simulink model "Doppelpendel_EKF_2015a"  (R2015a)
settings: Solver=ode45  StartTime=0.0  StopTime=10
undefined symbols (not defined in the file or in its folder): parDP, parEKF, parLQR
libraries: cstblocks x3
(part 2 of 2)

== matlab function Doppelpendel_EKF_2015a/Regler/LQR+EKF ==
  settings: updateMethod=DISCRETE  sampleTime=parLQR.Ta
  data: Switch_Rueckfuehrung input; statesd input; states input; uFF input; uG output; parDP parameter; parLQR parameter; parEKF parameter; xestout output; e_phi1 output; e_s output; e output; Pplus output
function [uG,xestout,e_phi1,e_s,e,Pplus]  = LQG(Switch_Rueckfuehrung,statesd,states,uFF,parDP,parLQR,parEKF)

%Anfangsbedinungen = Ruhelagen
persistent xI
if isempty(xI)
    xI = double(0);
end

persistent xminus
if isempty(xminus)
    xminus = [parEKF.phi10;parEKF.omega10;parEKF.phi20;parEKF.omega20;parEKF.s0;parEKF.w0];
end

persistent Pminus
if isempty( Pminus) 
    Pminus = diag([parEKF.delta,parEKF.delta,parEKF.delta,parEKF.delta,parEKF.delta,parEKF.delta]); 
end

%Ausgang
xestout=xminus;

%Beobachterrückführung ein/aus
if (Switch_Rueckfuehrung)
    xest=xestout;
else
    xest=states;
end

%%%%%%%%%%%%%%%%%%%%%%%%%%%%%%%%%%%%%%%%%%%%%%%%%%%%%%%%%%%%%%%%%%%%%%%%%%%
%LQR-Regler
%%%%%%%%%%%%%%%%%%%%%%%%%%%%%%%%%%%%%%%%%%%%%%%%%%%%%%%%%%%%%%%%%%%%%%%%%%%

% Folgendes hier bitte ausführen:
% 1.) PI-Zustandsregler einfügen

% xI(k+1) = xI(k) + (yd - y) (xI = eI)
xI = xI + (statesd(5) - xest(5));


% 2.) if (reset_cont==1) xI=0 end
% if (reset_cont==1)
%     xI=0;
% end

%Gesamtrückführung
% uFB = [kxT kI] [delta_e; delta_eI] (2.26b)
uG = parLQR.kx*(xest - statesd) + parLQR.kI * xI + uFF;

%%%%%%%%%%%%%%%%%%%%%%%%%%%%%%%%%%%%%%%%%%%%%%%%%%%%%%%%%%%%%%%%%%%%%%%%%%%
%EKF
%%%%%%%%%%%%%%%%%%%%%%%%%%%%%%%%%%%%%%%%%%%%%%%%%%%%%%%%%%%%%%%%%%%%%%%%%%%

% Folgendes hier bitte ausführen:
% 1.) Extended-Kalman-Filter einfügen

Ck = [0 0 0 0 1 0; 1 0 0 0 0 0];
% Hk = 0;
Lk_dach = Pminus*Ck' / (Ck*Pminus*Ck' + parEKF.Rn);

xplus = xminus + Lk_dach*( [states(5); states(1)] - [ xest(5); xest(1)] );
Pplus = (eye(6) - Lk_dach*Ck) * Pminus;

Phi_k = eye(6) + parDP.Ta*fcnAsys(xplus,uG,parDP);
Gk = eye(6);

xminus = xplus + parDP.Ta*fcnfx(xplus,uG,parDP);
Pminus = Phi_k*Pplus*Phi_k' + Gk*parEKF.Qn*Gk';

e_phi1 = states(1) - xminus(1);
e_s = states(5)- xminus(5);
e = 0;

end

%% Rechte Seite
function fx = fcnfx(xplus,uG,parDP)

InvD11 = parDP.m2*parDP.a2*parDP.a2+parDP.J2;
InvD12 = -parDP.m2*parDP.l1*parDP.a2*cos(xplus(1)-xplus(3));
InvD22 = parDP.J1+parDP.a1*parDP.a1*parDP.m1+parDP.m2*parDP.l1*parDP.l1;
den    = (parDP.J1+parDP.a1*parDP.a1*parDP.m1+parDP.m2*parDP.l1*parDP.l1)*(parDP.m2*parDP.a2*parDP.a2+parDP.J2)-parDP.m2*parDP.m2*parDP.l1*parDP.l1*parDP.a2*parDP.a2*(cos(xplus(1)-xplus(3)))^2;
gg1    = parDP.d2*xplus(2)-parDP.d2*xplus(4)-parDP.m2*parDP.l1*cos(xplus(1))*uG-parDP.m1*parDP.g*parDP.a1*sin(xplus(1))-parDP.m2*parDP.g*parDP.l1*sin(xplus(1))-parDP.m1*parDP.a1*cos(xplus(1))*uG+parDP.d1*xplus(2)+parDP.m2*parDP.l1*parDP.a2*xplus(4)*xplus(4)*sin(xplus(1)-xplus(3));
gg2    = -parDP.m2*parDP.g*parDP.a2*sin(xplus(3))-parDP.m2*parDP.a2*cos(xplus(3))*uG-parDP.m2*parDP.a2*parDP.l1*xplus(2)*xplus(2)*sin(xplus(1)-xplus(3))+parDP.d2*xplus(4)-parDP.d2*xplus(2);

fx = [xplus(2);
    -1/den*(InvD11*gg1+InvD12*gg2);
    xplus(4);
    -1/den*(InvD12*gg1+InvD22*gg2);
    xplus(6);
    uG];

end
%% linearisierte Systemmatrix

function Asyslin = fcnAsys(xplus,u,parDP) %% linearisierte Systemmatrix

Asyslin = [0 1 0 0 0 0;
    -0.1e1 / (parDP.J1 * parDP.m2 * parDP.a2 ^ 2 + parDP.J1 * parDP.J2 + parDP.a1 ^ 2 * parDP.m1 * parDP.m2 * parDP.a2 ^ 2 + parDP.a1 ^ 2 * parDP.m1 * parDP.J2 + parDP.m2 ^ 2 * parDP.l1 ^ 2 * parDP.a2 ^ 2 + parDP.m2 * parDP.l1 ^ 2 * parDP.J2 - parDP.m2 ^ 2 * parDP.l1 ^ 2 * parDP.a2 ^ 2 * cos(xplus(1)) ^ 2 * cos(xplus(3)) ^ 2 - 0.2e1 * parDP.m2 ^ 2 * parDP.l1 ^ 2 * parDP.a2 ^ 2 * cos(xplus(1)) * cos(xplus(3)) * sin(xplus(1)) * sin(xplus(3)) - parDP.m2 ^ 2 * parDP.l1 ^ 2 * parDP.a2 ^ 2 * sin(xplus(1)) ^ 2 * sin(xplus(3)) ^ 2) ^ 2 * (-parDP.d2 * xplus(2) * parDP.m2 * parDP.a2 ^ 2 + parDP.d2 * xplus(4) * parDP.m2 * parDP.a2 ^ 2 - parDP.d1 * xplus(2) * parDP.m2 * parDP.a2 ^ 2 + parDP.m2 ^ 2 * parDP.a2 ^ 3 * sin(xplus(3)) * xplus(4) * parDP.l1 * cos(xplus(1)) * xplus(2) - parDP.m2 ^ 2 * parDP.a2 ^ 3 * cos(xplus(3)) * xplus(4) * parDP.l1 * sin(xplus(1)) * xplus(2) + parDP.m1 * parDP.a1 * sin(xplus(1)) * xplus(2) * xplus(6) * parDP.m2 * parDP.a2 ^ 2 - parDP.m2 ^ 2 * parDP.l1 * parDP.a2 ^ 2 * cos(xplus(1)) * cos(xplus(3)) * parDP.g * sin(xplus(3)) - parDP.m2 ^ 2 * parDP.l1 * parDP.a2 ^ 2 * sin(xplus(1)) * sin(xplus(3)) ^ 2 * xplus(4) * xplus(6) - parDP.m2 ^ 2 * parDP.l1 * parDP.a2 ^ 2 * sin(xplus(1)) * sin(xplus(3)) * cos(xplus(3)) * u + parDP.m2 * parDP.l1 * parDP.a2 * cos(xplus(1)) * cos(xplus(3)) * parDP.d2 * xplus(4) - parDP.m2 * parDP.l1 * parDP.a2 * cos(xplus(1)) * cos(xplus(3)) * parDP.d2 * xplus(2) + parDP.m2 * parDP.l1 * parDP.a2 * sin(xplus(1)) * sin(xplus(3)) * parDP.d2 * xplus(4) - parDP.m2 * parDP.l1 * parDP.a2 * sin(xplus(1)) * sin(xplus(3)) * parDP.d2 * xplus(2) + parDP.m2 ^ 2 * parDP.l1 * cos(xplus(1)) * u * parDP.a2 ^ 2 + parDP.m2 * parDP.l1 * cos(xplus(1)) * u * parDP.J2 + parDP.m1 * parDP.g * parDP.a1 * sin(xplus(1)) * parDP.J2 + parDP.m2 ^ 2 * parDP.g * parDP.l1 * sin(xplus(1)) * parDP.a2 ^ 2 + parDP.m2 * parDP.g * parDP.l1 * sin(xplus(1)) * parDP.J2 + parDP.m1 * parDP.a1 * cos(xplus(1)) * u * parDP.J2 + parDP.m1 * parDP.g * parDP.a1 * sin(xplus(1)) * parDP.m2 * parDP.a2 ^ 2 + parDP.m1 * parDP.a1 * cos(xplus(1)) * u * parDP.m2 * parDP.a2 ^ 2 + parDP.m1 * parDP.a1 * sin(xplus(1)) * xplus(2) * xplus(6) * parDP.J2 + parDP.m2 ^ 2 * parDP.l1 * sin(xplus(1)) * xplus(2) * xplus(6) * parDP.a2 ^ 2 + parDP.m2 * parDP.l1 * sin(xplus(1)) * xplus(2) * xplus(6) * parDP.J2 - parDP.m2 ^ 2 * parDP.l1 * parDP.a2 ^ 2 * cos(xplus(1)) * cos(xplus(3)) ^ 2 * u - parDP.m2 ^ 2 * parDP.l1 * parDP.a2 ^ 2 * sin(xplus(1)) * sin(xplus(3)) ^ 2 * parDP.g - parDP.d2 * xplus(2) * parDP.J2 - parDP.d1 * xplus(2) * parDP.J2 + parDP.d2 * xplus(4) * parDP.J2 + parDP.m2 ^ 2 * parDP.l1 ^ 2 * parDP.a2 ^ 2 * cos(xplus(1)) ^ 2 * cos(xplus(3)) * sin(xplus(3)) * xplus(4) * xplus(2) + parDP.m2 ^ 2 * parDP.l1 ^ 2 * parDP.a2 ^ 2 * sin(xplus(1)) * sin(xplus(3)) ^ 2 * xplus(4) * cos(xplus(1)) * xplus(2) - parDP.m2 ^ 2 * parDP.l1 ^ 2 * parDP.a2 ^ 2 * sin(xplus(1)) ^ 2 * sin(xplus(3)) * cos(xplus(3)) * xplus(4) * xplus(2) - parDP.m2 ^ 2 * parDP.l1 ^ 2 * parDP.a2 ^ 2 * cos(xplus(1)) * cos(xplus(3)) ^ 2 * xplus(4) * sin(xplus(1)) * xplus(2) + parDP.m2 * parDP.a2 * sin(xplus(3)) * xplus(4) * parDP.l1 * cos(xplus(1)) * xplus(2) * parDP.J2 - parDP.m2 * parDP.a2 * cos(xplus(3)) * xplus(4) * parDP.l1 * sin(xplus(1)) * xplus(2) * parDP.J2 - parDP.m2 ^ 2 * parDP.l1 * parDP.a2 ^ 2 * cos(xplus(1)) * cos(xplus(3)) * sin(xplus(3)) * xplus(4) * xplus(6)) * (0.2e1 * parDP.m2 ^ 2 * parDP.l1 ^ 2 * parDP.a2 ^ 2 * cos(xplus(1)) * cos(xplus(3)) ^ 2 * sin(xplus(1)) + 0.2e1 * parDP.m2 ^ 2 * parDP.l1 ^ 2 * parDP.a2 ^ 2 * sin(xplus(1)) ^ 2 * cos(xplus(3)) * sin(xplus(3)) - 0.2e1 * parDP.m2 ^ 2 * parDP.l1 ^ 2 * parDP.a2 ^ 2 * cos(xplus(1)) ^ 2 * cos(xplus(3)) * sin(xplus(3)) - 0.2e1 * parDP.m2 ^ 2 * parDP.l1 ^ 2 * parDP.a2 ^ 2 * sin(xplus(1)) * sin(xplus(3)) ^ 2 * cos(xplus(1))) + 0.1e1 / (parDP.J1 * parDP.m2 * parDP.a2 ^ 2 + parDP.J1 * parDP.J2 + parDP.a1 ^ 2 * parDP.m1 * parDP.m2 * parDP.a2 ^ 2 + parDP.a1 ^ 2 * parDP.m1 * parDP.J2 + parDP.m2 ^ 2 * parDP.l1 ^ 2 * parDP.a2 ^ 2 + parDP.m2 * parDP.l1 ^ 2 * parDP.J2 - parDP.m2 ^ 2 * parDP.l1 ^ 2 * parDP.a2 ^ 2 * cos(xplus(1)) ^ 2 * cos(xplus(3)) ^ 2 - 0.2e1 * parDP.m2 ^ 2 * parDP.l1 ^ 2 * parDP.a2 ^ 2 * cos(xplus(1)) * cos(xplus(3)) * sin(xplus(1)) * sin(xplus(3)) - parDP.m2 ^ 2 * parDP.l1 ^ 2 * parDP.a2 ^ 2 * sin(xplus(1)) ^ 2 * sin(xplus(3)) ^ 2) * (-parDP.m2 ^ 2 * parDP.a2 ^ 3 * sin(xplus(3)) * xplus(4) * parDP.l1 * sin(xplus(1)) * xplus(2) - parDP.m2 ^ 2 * parDP.a2 ^ 3 * cos(xplus(3)) * xplus(4) * parDP.l1 * cos(xplus(1)) * xplus(2) + parDP.m1 * parDP.a1 * cos(xplus(1)) * xplus(2) * xplus(6) * parDP.m2 * parDP.a2 ^ 2 + parDP.m2 ^ 2 * parDP.l1 * parDP.a2 ^ 2 * sin(xplus(1)) * cos(xplus(3)) * parDP.g * sin(xplus(3)) - parDP.m2 ^ 2 * parDP.l1 * parDP.a2 ^ 2 * cos(xplus(1)) * sin(xplus(3)) ^ 2 * xplus(4) * xplus(6) - parDP.m2 ^ 2 * parDP.l1 * sin(xplus(1)) * u * parDP.a2 ^ 2 - parDP.m2 ^ 2 * parDP.l1 * parDP.a2 ^ 2 * cos(xplus(1)) * sin(xplus(3)) * cos(xplus(3)) * u - parDP.m2 * parDP.l1 * parDP.a2 * sin(xplus(1)) * cos(xplus(3)) * parDP.d2 * xplus(4) + parDP.m2 * parDP.l1 * parDP.a2 * sin(xplus(1)) * cos(xplus(3)) * parDP.d2 * xplus(2) + parDP.m2 * parDP.l1 * parDP.a2 * cos(xplus(1)) * sin(xplus(3)) * parDP.d2 * xplus(4) - parDP.m2 * parDP.l1 * parDP.a2 * cos(xplus(1)) * sin(xplus(3)) * parDP.d2 * xplus(2) - parDP.m2 ^ 2 * parDP.l1 ^ 2 * parDP.a2 ^ 2 * sin(xplus(1)) ^ 2 * sin(xplus(3)) ^ 2 * xplus(4) * xplus(2) + parDP.m2 ^ 2 * parDP.l1 ^ 2 * parDP.a2 ^ 2 * sin(xplus(1)) ^ 2 * cos(xplus(3)) ^ 2 * xplus(4) * xplus(2) + parDP.m1 * parDP.g * parDP.a1 * cos(xplus(1)) * parDP.m2 * parDP.a2 ^ 2 - parDP.m1 * parDP.a1 * sin(xplus(1)) * u * parDP.m2 * parDP.a2 ^ 2 + parDP.m1 * parDP.a1 * cos(xplus(1)) * xplus(2) * xplus(6) * parDP.J2 + parDP.m2 ^ 2 * parDP.l1 * cos(xplus(1)) * xplus(2) * xplus(6) * parDP.a2 ^ 2 + parDP.m2 * parDP.l1 * cos(xplus(1)) * xplus(2) * xplus(6) * parDP.J2 + parDP.m2 ^ 2 * parDP.l1 * parDP.a2 ^ 2 * sin(xplus(1)) * cos(xplus(3)) ^ 2 * u - parDP.m2 ^ 2 * parDP.l1 * parDP.a2 ^ 2 * cos(xplus(1)) * sin(xplus(3)) ^ 2 * parDP.g - parDP.m2 * parDP.l1 * sin(xplus(1)) * u * parDP.J2 + parDP.m1 * parDP.g * parDP.a1 * cos(xplus(1)) * parDP.J2 + parDP.m2 ^ 2 * parDP.g * parDP.l1 * cos(xplus(1)) * parDP.a2 ^ 2 + parDP.m2 * parDP.g * parDP.l1 * cos(xplus(1)) * parDP.J2 - parDP.m1 * parDP.a1 * sin(xplus(1)) * u * parDP.J2 - 0.4e1 * parDP.m2 ^ 2 * parDP.l1 ^ 2 * parDP.a2 ^ 2 * cos(xplus(1)) * cos(xplus(3)) * sin(xplus(3)) * xplus(4) * xplus(2) * sin(xplus(1)) + parDP.m2 ^ 2 * parDP.l1 ^ 2 * parDP.a2 ^ 2 * cos(xplus(1)) ^ 2 * sin(xplus(3)) ^ 2 * xplus(4) * xplus(2) - parDP.m2 ^ 2 * parDP.l1 ^ 2 * parDP.a2 ^ 2 * cos(xplus(1)) ^ 2 * cos(xplus(3)) ^ 2 * xplus(4) * xplus(2) - parDP.m2 * parDP.a2 * sin(xplus(3)) * xplus(4) * parDP.l1 * sin(xplus(1)) * xplus(2) * parDP.J2 - parDP.m2 * parDP.a2 * cos(xplus(3)) * xplus(4) * parDP.l1 * cos(xplus(1)) * xplus(2) * parDP.J2 + parDP.m2 ^ 2 * parDP.l1 * parDP.a2 ^ 2 * sin(xplus(1)) * cos(xplus(3)) * sin(xplus(3)) * xplus(4) * xplus(6)) 0.1e1 / (parDP.J1 * parDP.m2 * parDP.a2 ^ 2 + parDP.J1 * parDP.J2 + parDP.a1 ^ 2 * parDP.m1 * parDP.m2 * parDP.a2 ^ 2 + parDP.a1 ^ 2 * parDP.m1 * parDP.J2 + parDP.m2 ^ 2 * parDP.l1 ^ 2 * parDP.a2 ^ 2 + parDP.m2 * parDP.l1 ^ 2 * parDP.J2 - parDP.m2 ^ 2 * parDP.l1 ^ 2 * parDP.a2 ^ 2 * cos(xplus(1)) ^ 2 * cos(xplus(3)) ^ 2 - 0.2e1 * parDP.m2 ^ 2 * parDP.l1 ^ 2 * parDP.a2 ^ 2 * cos(xplus(1)) * cos(xplus(3)) * sin(xplus(1)) * sin(xplus(3)) - parDP.m2 ^ 2 * parDP.l1 ^ 2 * parDP.a2 ^ 2 * sin(xplus(1)) ^ 2 * sin(xplus(3)) ^ 2) * (-parDP.d2 * parDP.m2 * parDP.a2 ^ 2 - parDP.d1 * parDP.m2 * parDP.a2 ^ 2 + parDP.m2 ^ 2 * parDP.a2 ^ 3 * sin(xplus(3)) * xplus(4) * parDP.l1 * cos(xplus(1)) - parDP.m2 ^ 2 * parDP.a2 ^ 3 * cos(xplus(3)) * xplus(4) * parDP.l1 * sin(xplus(1)) + parDP.m1 * parDP.a1 * sin(xplus(1)) * xplus(6) * parDP.m2 * parDP.a2 ^ 2 - parDP.m2 * parDP.l1 * parDP.a2 * cos(xplus(1)) * cos(xplus(3)) * parDP.d2 - parDP.m2 * parDP.l1 * parDP.a2 * sin(xplus(1)) * sin(xplus(3)) * parDP.d2 + parDP.m1 * parDP.a1 * sin(xplus(1)) * xplus(6) * parDP.J2 + parDP.m2 ^ 2 * parDP.l1 * sin(xplus(1)) * xplus(6) * parDP.a2 ^ 2 + parDP.m2 * parDP.l1 * sin(xplus(1)) * xplus(6) * parDP.J2 - parDP.d2 * parDP.J2 - parDP.d1 * parDP.J2 + parDP.m2 ^ 2 * parDP.l1 ^ 2 * parDP.a2 ^ 2 * cos(xplus(1)) ^ 2 * cos(xplus(3)) * sin(xplus(3)) * xplus(4) + parDP.m2 ^ 2 * parDP.l1 ^ 2 * parDP.a2 ^ 2 * sin(xplus(1)) * sin(xplus(3)) ^ 2 * xplus(4) * cos(xplus(1)) - parDP.m2 ^ 2 * parDP.l1 ^ 2 * parDP.a2 ^ 2 * sin(xplus(1)) ^ 2 * sin(xplus(3)) * cos(xplus(3)) * xplus(4) - parDP.m2 ^ 2 * parDP.l1 ^ 2 * parDP.a2 ^ 2 * cos(xplus(1)) * cos(xplus(3)) ^ 2 * xplus(4) * sin(xplus(1)) + parDP.m2 * parDP.a2 * sin(xplus(3)) * xplus(4) * parDP.l1 * cos(xplus(1)) * parDP.J2 - parDP.m2 * parDP.a2 * cos(xplus(3)) * xplus(4) * parDP.l1 * sin(xplus(1)) * parDP.J2) -0.1e1 / (parDP.J1 * parDP.m2 * parDP.a2 ^ 2 + parDP.J1 * parDP.J2 + parDP.a1 ^ 2 * parDP.m1 * parDP.m2 * parDP.a2 ^ 2 + parDP.a1 ^ 2 * parDP.m1 * parDP.J2 + parDP.m2 ^ 2 * parDP.l1 ^ 2 * parDP.a2 ^ 2 + parDP.m2 * parDP.l1 ^ 2 * parDP.J2 - parDP.m2 ^ 2 * parDP.l1 ^ 2 * parDP.a2 ^ 2 * cos(xplus(1)) ^ 2 * cos(xplus(3)) ^ 2 - 0.2e1 * parDP.m2 ^ 2 * parDP.l1 ^ 2 * parDP.a2 ^ 2 * cos(xplus(1)) * cos(xplus(3)) * sin(xplus(1)) * sin(xplus(3)) - parDP.m2 ^ 2 * parDP.l1 ^ 2 * parDP.a2 ^ 2 * sin(xplus(1)) ^ 2 * sin(xplus(3)) ^ 2) ^ 2 * (-parDP.d2 * xplus(2) * parDP.m2 * parDP.a2 ^ 2 + parDP.d2 * xplus(4) * parDP.m2 * parDP.a2 ^ 2 - parDP.d1 * xplus(2) * parDP.m2 * parDP.a2 ^ 2 + parDP.m2 ^ 2 * parDP.a2 ^ 3 * sin(xplus(3)) * xplus(4) * parDP.l1 * cos(xplus(1)) * xplus(2) - parDP.m2 ^ 2 * parDP.a2 ^ 3 * cos(xplus(3)) * xplus(4) * parDP.l1 * sin(xplus(1)) * xplus(2) + parDP.m1 * parDP.a1 * sin(xplus(1)) * xplus(2) * xplus(6) * parDP.m2 * parDP.a2 ^ 2 - parDP.m2 ^ 2 * parDP.l1 * parDP.a2 ^ 2 * cos(xplus(1)) * cos(xplus(3)) * parDP.g * sin(xplus(3)) - parDP.m2 ^ 2 * parDP.l1 * parDP.a2 ^ 2 * sin(xplus(1)) * sin(xplus(3)) ^ 2 * xplus(4) * xplus(6) - parDP.m2 ^ 2 * parDP.l1 * parDP.a2 ^ 2 * sin(xplus(1)) * sin(xplus(3)) * cos(xplus(3)) * u + parDP.m2 * parDP.l1 * parDP.a2 * cos(xplus(1)) * cos(xplus(3)) * parDP.d2 * xplus(4) - parDP.m2 * parDP.l1 * parDP.a2 * cos(xplus(1)) * cos(xplus(3)) * parDP.d2 * xplus(2) + parDP.m2 * parDP.l1 * parDP.a2 * sin(xplus(1)) * sin(xplus(3)) * parDP.d2 * xplus(4) - parDP.m2 * parDP.l1 * parDP.a2 * sin(xplus(1)) * sin(xplus(3)) * parDP.d2 * xplus(2) + parDP.m2 ^ 2 * parDP.l1 * cos(xplus(1)) * u * parDP.a2 ^ 2 + parDP.m2 * parDP.l1 * cos(xplus(1)) * u * parDP.J2 + parDP.m1 * parDP.g * parDP.a1 * sin(xplus(1)) * parDP.J2 + parDP.m2 ^ 2 * parDP.g * parDP.l1 * sin(xplus(1)) * parDP.a2 ^ 2 + parDP.m2 * parDP.g * parDP.l1 * sin(xplus(1)) * parDP.J2 + parDP.m1 * parDP.a1 * cos(xplus(1)) * u * parDP.J2 + parDP.m1 * parDP.g * parDP.a1 * sin(xplus(1)) * parDP.m2 * parDP.a2 ^ 2 + parDP.m1 * parDP.a1 * cos(xplus(1)) * u * parDP.m2 * parDP.a2 ^ 2 + parDP.m1 * parDP.a1 * sin(xplus(1)) * xplus(2) * xplus(6) * parDP.J2 + parDP.m2 ^ 2 * parDP.l1 * sin(xplus(1)) * xplus(2) * xplus(6) * parDP.a2 ^ 2 + parDP.m2 * parDP.l1 * sin(xplus(1)) * xplus(2) * xplus(6) * parDP.J2 - parDP.m2 ^ 2 * parDP.l1 * parDP.a2 ^ 2 * cos(xplus(1)) * cos(xplus(3)) ^ 2 * u - parDP.m2 ^ 2 * parDP.l1 * parDP.a2 ^ 2 * sin(xplus(1)) * sin(xplus(3)) ^ 2 * parDP.g - parDP.d2 * xplus(2) * parDP.J2 - parDP.d1 * xplus(2) * parDP.J2 + parDP.d2 * xplus(4) * parDP.J2 + parDP.m2 ^ 2 * parDP.l1 ^ 2 * parDP.a2 ^ 2 * cos(xplus(1)) ^ 2 * cos(xplus(3)) * sin(xplus(3)) * xplus(4) * xplus(2) + parDP.m2 ^ 2 * parDP.l1 ^ 2 * parDP.a2 ^ 2 * sin(xplus(1)) * sin(xplus(3)) ^ 2 * xplus(4) * cos(xplus(1)) * xplus(2) - parDP.m2 ^ 2 * parDP.l1 ^ 2 * parDP.a2 ^ 2 * sin(xplus(1)) ^ 2 * sin(xplus(3)) * cos(xplus(3)) * xplus(4) * xplus(2) - parDP.m2 ^ 2 * parDP.l1 ^ 2 * parDP.a2 ^ 2 * cos(xplus(1)) * cos(xplus(3)) ^ 2 * xplus(4) * sin(xplus(1)) * xplus(2) + parDP.m2 * parDP.a2 * sin(xplus(3)) * xplus(4) * parDP.l1 * cos(xplus(1)) * xplus(2) * parDP.J2 - parDP.m2 * parDP.a2 * cos(xplus(3)) * xplus(4) * parDP.l1 * sin(xplus(1)) * xplus(2) * parDP.J2 - parDP.m2 ^ 2 * parDP.l1 * parDP.a2 ^ 2 * cos(xplus(1)) * cos(xplus(3)) * sin(xplus(3)) * xplus(4) * xplus(6)) * (0.2e1 * parDP.m2 ^ 2 * parDP.l1 ^ 2 * parDP.a2 ^ 2 * cos(xplus(1)) ^ 2 * cos(xplus(3)) * sin(xplus(3)) + 0.2e1 * parDP.m2 ^ 2 * parDP.l1 ^ 2 * parDP.a2 ^ 2 * sin(xplus(1)) * sin(xplus(3)) ^ 2 * cos(xplus(1)) - 0.2e1 * parDP.m2 ^ 2 * parDP.l1 ^ 2 * parDP.a2 ^ 2 * cos(xplus(1)) * cos(xplus(3)) ^ 2 * sin(xplus(1)) - 0.2e1 * parDP.m2 ^ 2 * parDP.l1 ^ 2 * parDP.a2 ^ 2 * sin(xplus(1)) ^ 2 * cos(xplus(3)) * sin(xplus(3))) + 0.1e1 / (parDP.J1 * parDP.m2 * parDP.a2 ^ 2 + parDP.J1 * parDP.J2 + parDP.a1 ^ 2 * parDP.m1 * parDP.m2 * parDP.a2 ^ 2 + parDP.a1 ^ 2 * parDP.m1 * parDP.J2 + parDP.m2 ^ 2 * parDP.l1 ^ 2 * parDP.a2 ^ 2 + parDP.m2 * parDP.l1 ^ 2 * parDP.J2 - parDP.m2 ^ 2 * parDP.l1 ^ 2 * parDP.a2 ^ 2 * cos(xplus(1)) ^ 2 * cos(xplus(3)) ^ 2 - 0.2e1 * parDP.m2 ^ 2 * parDP.l1 ^ 2 * parDP.a2 ^ 2 * cos(xplus(1)) * cos(xplus(3)) * sin(xplus(1)) * sin(xplus(3)) - parDP.m2 ^ 2 * parDP.l1 ^ 2 * parDP.a2 ^ 2 * sin(xplus(1)) ^ 2 * sin(xplus(3)) ^ 2) * (parDP.m2 ^ 2 * parDP.a2 ^ 3 * cos(xplus(3)) * xplus(4) * parDP.l1 * cos(xplus(1)) * xplus(2) + parDP.m2 ^ 2 * parDP.a2 ^ 3 * sin(xplus(3)) * xplus(4) * parDP.l1 * sin(xplus(1)) * xplus(2) + parDP.m2 ^ 2 * parDP.l1 * parDP.a2 ^ 2 * cos(xplus(1)) * sin(xplus(3)) ^ 2 * parDP.g - parDP.m2 ^ 2 * parDP.l1 * parDP.a2 ^ 2 * cos(xplus(1)) * cos(xplus(3)) ^ 2 * parDP.g - 0.2e1 * parDP.m2 ^ 2 * parDP.l1 * parDP.a2 ^ 2 * sin(xplus(1)) * cos(xplus(3)) * sin(xplus(3)) * xplus(4) * xplus(6) - parDP.m2 ^ 2 * parDP.l1 * parDP.a2 ^ 2 * sin(xplus(1)) * cos(xplus(3)) ^ 2 * u + parDP.m2 ^ 2 * parDP.l1 * parDP.a2 ^ 2 * sin(xplus(1)) * sin(xplus(3)) ^ 2 * u - parDP.m2 * parDP.l1 * parDP.a2 * cos(xplus(1)) * sin(xplus(3)) * parDP.d2 * xplus(4) + parDP.m2 * parDP.l1 * parDP.a2 * cos(xplus(1)) * sin(xplus(3)) * parDP.d2 * xplus(2) + parDP.m2 * parDP.l1 * parDP.a2 * sin(xplus(1)) * cos(xplus(3)) * parDP.d2 * xplus(4) - parDP.m2 * parDP.l1 * parDP.a2 * sin(xplus(1)) * cos(xplus(3)) * parDP.d2 * xplus(2) + 0.2e1 * parDP.m2 ^ 2 * parDP.l1 * parDP.a2 ^ 2 * cos(xplus(1)) * sin(xplus(3)) * cos(xplus(3)) * u - 0.2e1 * parDP.m2 ^ 2 * parDP.l1 * parDP.a2 ^ 2 * sin(xplus(1)) * cos(xplus(3)) * parDP.g * sin(xplus(3)) - parDP.m2 ^ 2 * parDP.l1 ^ 2 * parDP.a2 ^ 2 * cos(xplus(1)) ^ 2 * sin(xplus(3)) ^ 2 * xplus(4) * xplus(2) + parDP.m2 ^ 2 * parDP.l1 ^ 2 * parDP.a2 ^ 2 * cos(xplus(1)) ^ 2 * cos(xplus(3)) ^ 2 * xplus(4) * xplus(2) + 0.4e1 * parDP.m2 ^ 2 * parDP.l1 ^ 2 * parDP.a2 ^ 2 * cos(xplus(1)) * cos(xplus(3)) * sin(xplus(3)) * xplus(4) * xplus(2) * sin(xplus(1)) - parDP.m2 ^ 2 * parDP.l1 ^ 2 * parDP.a2 ^ 2 * sin(xplus(1)) ^ 2 * cos(xplus(3)) ^ 2 * xplus(4) * xplus(2) + parDP.m2 ^ 2 * parDP.l1 ^ 2 * parDP.a2 ^ 2 * sin(xplus(1)) ^ 2 * sin(xplus(3)) ^ 2 * xplus(4) * xplus(2) + parDP.m2 * parDP.a2 * cos(xplus(3)) * xplus(4) * parDP.l1 * cos(xplus(1)) * xplus(2) * parDP.J2 + parDP.m2 * parDP.a2 * sin(xplus(3)) * xplus(4) * parDP.l1 * sin(xplus(1)) * xplus(2) * parDP.J2 + parDP.m2 ^ 2 * parDP.l1 * parDP.a2 ^ 2 * cos(xplus(1)) * sin(xplus(3)) ^ 2 * xplus(4) * xplus(6) - parDP.m2 ^ 2 * parDP.l1 * parDP.a2 ^ 2 * cos(xplus(1)) * cos(xplus(3)) ^ 2 * xplus(4) * xplus(6)) 0.1e1 / (parDP.J1 * parDP.m2 * parDP.a2 ^ 2 + parDP.J1 * parDP.J2 + parDP.a1 ^ 2 * parDP.m1 * parDP.m2 * parDP.a2 ^ 2 + parDP.a1 ^ 2 * parDP.m1 * parDP.J2 + parDP.m2 ^ 2 * parDP.l1 ^ 2 * parDP.a2 ^ 2 + parDP.m2 * parDP.l1 ^ 2 * parDP.J2 - parDP.m2 ^ 2 * parDP.l1 ^ 2 * parDP.a2 ^ 2 * cos(xplus(1)) ^ 2 * cos(xplus(3)) ^ 2 - 0.2e1 * parDP.m2 ^ 2 * parDP.l1 ^ 2 * parDP.a2 ^ 2 * cos(xplus(1)) * cos(xplus(3)) * sin(xplus(1)) * sin(xplus(3)) - parDP.m2 ^ 2 * parDP.l1 ^ 2 * parDP.a2 ^ 2 * sin(xplus(1)) ^ 2 * sin(xplus(3)) ^ 2) * (parDP.d2 * parDP.m2 * parDP.a2 ^ 2 + parDP.m2 ^ 2 * parDP.a2 ^ 3 * sin(xplus(3)) * parDP.l1 * cos(xplus(1)) * xplus(2) - parDP.m2 ^ 2 * parDP.a2 ^ 3 * cos(xplus(3)) * parDP.l1 * sin(xplus(1)) * xplus(2) - parDP.m2 ^ 2 * parDP.l1 * parDP.a2 ^ 2 * sin(xplus(1)) * sin(xplus(3)) ^ 2 * xplus(6) + parDP.m2 * parDP.l1 * parDP.a2 * cos(xplus(1)) * cos(xplus(3)) * parDP.d2 + parDP.m2 * parDP.l1 * parDP.a2 * sin(xplus(1)) * sin(xplus(3)) * parDP.d2 + parDP.d2 * parDP.J2 + parDP.m2 ^ 2 * parDP.l1 ^ 2 * parDP.a2 ^ 2 * cos(xplus(1)) ^ 2 * cos(xplus(3)) * sin(xplus(3)) * xplus(2) + parDP.m2 ^ 2 * parDP.l1 ^ 2 * parDP.a2 ^ 2 * sin(xplus(1)) * sin(xplus(3)) ^ 2 * cos(xplus(1)) * xplus(2) - parDP.m2 ^ 2 * parDP.l1 ^ 2 * parDP.a2 ^ 2 * sin(xplus(1)) ^ 2 * sin(xplus(3)) * cos(xplus(3)) * xplus(2) - parDP.m2 ^ 2 * parDP.l1 ^ 2 * parDP.a2 ^ 2 * cos(xplus(1)) * cos(xplus(3)) ^ 2 * sin(xplus(1)) * xplus(2) + parDP.m2 * parDP.a2 * sin(xplus(3)) * parDP.l1 * cos(xplus(1)) * xplus(2) * parDP.J2 - parDP.m2 * parDP.a2 * cos(xplus(3)) * parDP.l1 * sin(xplus(1)) * xplus(2) * parDP.J2 - parDP.m2 ^ 2 * parDP.l1 * parDP.a2 ^ 2 * cos(xplus(1)) * cos(xplus(3)) * sin(xplus(3)) * xplus(6)) 0 0.1e1 / (parDP.J1 * parDP.m2 * parDP.a2 ^ 2 + parDP.J1 * parDP.J2 + parDP.a1 ^ 2 * parDP.m1 * parDP.m2 * parDP.a2 ^ 2 + parDP.a1 ^ 2 * parDP.m1 * parDP.J2 + parDP.m2 ^ 2 * parDP.l1 ^ 2 * parDP.a2 ^ 2 + parDP.m2 * parDP.l1 ^ 2 * parDP.J2 - parDP.m2 ^ 2 * parDP.l1 ^ 2 * parDP.a2 ^ 2 * cos(xplus(1)) ^ 2 * cos(xplus(3)) ^ 2 - 0.2e1 * parDP.m2 ^ 2 * parDP.l1 ^ 2 * parDP.a2 ^ 2 * cos(xplus(1)) * cos(xplus(3)) * sin(xplus(1)) * sin(xplus(3)) - parDP.m2 ^ 2 * parDP.l1 ^ 2 * parDP.a2 ^ 2 * sin(xplus(1)) ^ 2 * sin(xplus(3)) ^ 2) * (parDP.m1 * parDP.a1 * sin(xplus(1)) * xplus(2) * parDP.m2 * parDP.a2 ^ 2 - parDP.m2 ^ 2 * parDP.l1 * parDP.a2 ^ 2 * sin(xplus(1)) * sin(xplus(3)) ^ 2 * xplus(4) + parDP.m1 * parDP.a1 * sin(xplus(1)) * xplus(2) * parDP.J2 + parDP.m2 ^ 2 * parDP.l1 * sin(xplus(1)) * xplus(2) * parDP.a2 ^ 2 + parDP.m2 * parDP.l1 * sin(xplus(1)) * xplus(2) * parDP.J2 - parDP.m2 ^ 2 * parDP.l1 * parDP.a2 ^ 2 * cos(xplus(1)) * cos(xplus(3)) * sin(xplus(3)) * xplus(4))     ;
    0 0 0 1 0 0;
    (parDP.m2 * parDP.l1 * parDP.a2 * sin(xplus(1)) * cos(xplus(3)) * parDP.d2 * xplus(4) - parDP.m2 * parDP.l1 * parDP.a2 * sin(xplus(1)) * cos(xplus(3)) * parDP.d2 * xplus(2) - parDP.m2 * parDP.l1 * parDP.a2 * cos(xplus(1)) * sin(xplus(3)) * parDP.d2 * xplus(4) + parDP.m2 * parDP.l1 * parDP.a2 * cos(xplus(1)) * sin(xplus(3)) * parDP.d2 * xplus(2) + parDP.m2 ^ 2 * parDP.l1 ^ 2 * parDP.a2 ^ 2 * sin(xplus(1)) ^ 2 * sin(xplus(3)) ^ 2 * xplus(4) * xplus(2) - parDP.m2 ^ 2 * parDP.l1 ^ 2 * parDP.a2 ^ 2 * sin(xplus(1)) ^ 2 * cos(xplus(3)) ^ 2 * xplus(4) * xplus(2) + parDP.m2 ^ 2 * parDP.l1 ^ 2 * parDP.a2 * sin(xplus(1)) ^ 2 * sin(xplus(3)) * u + 0.4e1 * parDP.m2 ^ 2 * parDP.l1 ^ 2 * parDP.a2 ^ 2 * cos(xplus(1)) * cos(xplus(3)) * sin(xplus(3)) * xplus(4) * xplus(2) * sin(xplus(1)) - parDP.m2 ^ 2 * parDP.l1 ^ 2 * parDP.a2 ^ 2 * cos(xplus(1)) ^ 2 * sin(xplus(3)) ^ 2 * xplus(4) * xplus(2) + parDP.m2 ^ 2 * parDP.l1 ^ 2 * parDP.a2 ^ 2 * cos(xplus(1)) ^ 2 * cos(xplus(3)) ^ 2 * xplus(4) * xplus(2) + parDP.m2 ^ 2 * parDP.a2 * sin(xplus(3)) * xplus(4) * parDP.l1 ^ 3 * sin(xplus(1)) * xplus(2) - parDP.m2 * parDP.l1 * parDP.a2 * sin(xplus(1)) * cos(xplus(3)) * parDP.d1 * xplus(2) + parDP.m2 * parDP.l1 * parDP.a2 * cos(xplus(1)) * sin(xplus(3)) * parDP.d1 * xplus(2) - parDP.m2 ^ 2 * parDP.l1 ^ 2 * parDP.a2 * cos(xplus(1)) ^ 2 * cos(xplus(3)) * parDP.g - parDP.m2 ^ 2 * parDP.l1 ^ 2 * parDP.a2 * cos(xplus(1)) ^ 2 * sin(xplus(3)) * u + parDP.m2 ^ 2 * parDP.a2 * cos(xplus(3)) * xplus(4) * parDP.l1 ^ 3 * cos(xplus(1)) * xplus(2) - 0.2e1 * parDP.m2 ^ 2 * parDP.l1 ^ 2 * parDP.a2 * sin(xplus(1)) * sin(xplus(3)) * parDP.g * cos(xplus(1)) + 0.2e1 * parDP.m2 ^ 2 * parDP.l1 ^ 2 * parDP.a2 * cos(xplus(1)) * cos(xplus(3)) * u * sin(xplus(1)) + parDP.m2 ^ 2 * parDP.l1 ^ 2 * parDP.a2 * sin(xplus(1)) ^ 2 * cos(xplus(3)) * parDP.g - 0.2e1 * parDP.m2 ^ 2 * parDP.l1 ^ 2 * parDP.a2 * sin(xplus(1)) * sin(xplus(3)) * xplus(2) * xplus(6) * cos(xplus(1)) + 0.2e1 * parDP.m2 * parDP.l1 * parDP.a2 * cos(xplus(1)) * cos(xplus(3)) * parDP.m1 * parDP.a1 * u * sin(xplus(1)) + parDP.m2 ^ 2 * parDP.l1 ^ 2 * parDP.a2 * sin(xplus(1)) ^ 2 * cos(xplus(3)) * xplus(2) * xplus(6) - parDP.m2 * parDP.l1 * parDP.a2 * cos(xplus(1)) ^ 2 * cos(xplus(3)) * parDP.m1 * parDP.a1 * xplus(2) * xplus(6) + parDP.m2 * parDP.l1 * parDP.a2 * sin(xplus(1)) ^ 2 * cos(xplus(3)) * parDP.m1 * parDP.a1 * xplus(2) * xplus(6) - 0.2e1 * parDP.m2 * parDP.l1 * parDP.a2 * sin(xplus(1)) * sin(xplus(3)) * parDP.m1 * parDP.g * parDP.a1 * cos(xplus(1)) - parDP.m2 ^ 2 * parDP.l1 ^ 2 * parDP.a2 * cos(xplus(1)) ^ 2 * cos(xplus(3)) * xplus(2) * xplus(6) - parDP.m2 * parDP.l1 * parDP.a2 * cos(xplus(1)) ^ 2 * cos(xplus(3)) * parDP.m1 * parDP.g * parDP.a1 + parDP.m2 * parDP.l1 * parDP.a2 * sin(xplus(1)) ^ 2 * cos(xplus(3)) * parDP.m1 * parDP.g * parDP.a1 - parDP.m2 * parDP.l1 * parDP.a2 * cos(xplus(1)) ^ 2 * sin(xplus(3)) * parDP.m1 * parDP.a1 * u + parDP.m2 * parDP.l1 * parDP.a2 * sin(xplus(1)) ^ 2 * sin(xplus(3)) * parDP.m1 * parDP.a1 * u - 0.2e1 * parDP.m2 * parDP.l1 * parDP.a2 * sin(xplus(1)) * sin(xplus(3)) * parDP.m1 * parDP.a1 * xplus(2) * xplus(6) * cos(xplus(1)) + parDP.m2 * parDP.a2 * sin(xplus(3)) * xplus(4) * parDP.l1 * sin(xplus(1)) * xplus(2) * parDP.J1 + parDP.m2 * parDP.a2 * sin(xplus(3)) * xplus(4) * parDP.l1 * sin(xplus(1)) * xplus(2) * parDP.a1 ^ 2 * parDP.m1 + parDP.m2 * parDP.a2 * cos(xplus(3)) * xplus(4) * parDP.l1 * cos(xplus(1)) * xplus(2) * parDP.J1 + parDP.m2 * parDP.a2 * cos(xplus(3)) * xplus(4) * parDP.l1 * cos(xplus(1)) * xplus(2) * parDP.a1 ^ 2 * parDP.m1) / (parDP.J1 * parDP.m2 * parDP.a2 ^ 2 + parDP.J1 * parDP.J2 + parDP.a1 ^ 2 * parDP.m1 * parDP.m2 * parDP.a2 ^ 2 + parDP.a1 ^ 2 * parDP.m1 * parDP.J2 + parDP.m2 ^ 2 * parDP.l1 ^ 2 * parDP.a2 ^ 2 + parDP.m2 * parDP.l1 ^ 2 * parDP.J2 - parDP.m2 ^ 2 * parDP.l1 ^ 2 * parDP.a2 ^ 2 * cos(xplus(1)) ^ 2 * cos(xplus(3)) ^ 2 - 0.2e1 * parDP.m2 ^ 2 * parDP.l1 ^ 2 * parDP.a2 ^ 2 * cos(xplus(1)) * cos(xplus(3)) * sin(xplus(1)) * sin(xplus(3)) - parDP.m2 ^ 2 * parDP.l1 ^ 2 * parDP.a2 ^ 2 * sin(xplus(1)) ^ 2 * sin(xplus(3)) ^ 2) - (parDP.d2 * xplus(2) * parDP.m2 * parDP.l1 ^ 2 - parDP.d2 * xplus(4) * parDP.m2 * parDP.l1 ^ 2 - parDP.d2 * xplus(4) * parDP.a1 ^ 2 * parDP.m1 + parDP.d2 * xplus(2) * parDP.a1 ^ 2 * parDP.m1 - parDP.m2 ^ 2 * parDP.a2 * sin(xplus(3)) * xplus(4) * parDP.l1 ^ 3 * cos(xplus(1)) * xplus(2) - parDP.m2 * parDP.l1 * parDP.a2 * cos(xplus(1)) * cos(xplus(3)) * parDP.d2 * xplus(4) + parDP.m2 * parDP.l1 * parDP.a2 * cos(xplus(1)) * cos(xplus(3)) * parDP.d2 * xplus(2) - parDP.m2 * parDP.l1 * parDP.a2 * sin(xplus(1)) * sin(xplus(3)) * parDP.d2 * xplus(4) + parDP.m2 * parDP.l1 * parDP.a2 * sin(xplus(1)) * sin(xplus(3)) * parDP.d2 * xplus(2) + parDP.m2 * parDP.l1 * parDP.a2 * cos(xplus(1)) * cos(xplus(3)) * parDP.d1 * xplus(2) + parDP.m2 * parDP.l1 * parDP.a2 * sin(xplus(1)) * sin(xplus(3)) * parDP.d1 * xplus(2) - parDP.m2 ^ 2 * parDP.l1 ^ 2 * parDP.a2 * cos(xplus(1)) * cos(xplus(3)) * parDP.g * sin(xplus(1)) - parDP.m2 ^ 2 * parDP.l1 ^ 2 * parDP.a2 * sin(xplus(1)) * sin(xplus(3)) * cos(xplus(1)) * u + parDP.m2 ^ 2 * parDP.a2 * cos(xplus(3)) * xplus(4) * parDP.l1 ^ 3 * sin(xplus(1)) * xplus(2) - parDP.m2 ^ 2 * parDP.l1 ^ 2 * parDP.a2 * sin(xplus(1)) ^ 2 * sin(xplus(3)) * xplus(2) * xplus(6) + parDP.m2 * parDP.a2 * sin(xplus(3)) * xplus(4) * xplus(6) * parDP.a1 ^ 2 * parDP.m1 + parDP.m2 ^ 2 * parDP.g * parDP.a2 * sin(xplus(3)) * parDP.l1 ^ 2 + parDP.m2 * parDP.g * parDP.a2 * sin(xplus(3)) * parDP.J1 + parDP.m2 * parDP.a2 * cos(xplus(3)) * u * parDP.J1 + parDP.m2 ^ 2 * parDP.a2 * cos(xplus(3)) * u * parDP.l1 ^ 2 - parDP.m2 ^ 2 * parDP.l1 ^ 2 * parDP.a2 * sin(xplus(1)) ^ 2 * sin(xplus(3)) * parDP.g + parDP.m2 * parDP.a2 * sin(xplus(3)) * xplus(4) * xplus(6) * parDP.J1 + parDP.m2 ^ 2 * parDP.a2 * sin(xplus(3)) * xplus(4) * xplus(6) * parDP.l1 ^ 2 + parDP.m2 * parDP.g * parDP.a2 * sin(xplus(3)) * parDP.a1 ^ 2 * parDP.m1 + parDP.m2 * parDP.a2 * cos(xplus(3)) * u * parDP.a1 ^ 2 * parDP.m1 - parDP.m2 ^ 2 * parDP.l1 ^ 2 * parDP.a2 * cos(xplus(1)) ^ 2 * cos(xplus(3)) * u - parDP.d2 * xplus(4) * parDP.J1 + parDP.d2 * xplus(2) * parDP.J1 - parDP.m2 ^ 2 * parDP.l1 ^ 2 * parDP.a2 ^ 2 * cos(xplus(1)) ^ 2 * cos(xplus(3)) * sin(xplus(3)) * xplus(4) * xplus(2) - parDP.m2 ^ 2 * parDP.l1 ^ 2 * parDP.a2 ^ 2 * sin(xplus(1)) * sin(xplus(3)) ^ 2 * xplus(4) * cos(xplus(1)) * xplus(2) + parDP.m2 ^ 2 * parDP.l1 ^ 2 * parDP.a2 ^ 2 * sin(xplus(1)) ^ 2 * sin(xplus(3)) * cos(xplus(3)) * xplus(4) * xplus(2) + parDP.m2 ^ 2 * parDP.l1 ^ 2 * parDP.a2 ^ 2 * cos(xplus(1)) * cos(xplus(3)) ^ 2 * xplus(4) * sin(xplus(1)) * xplus(2) - parDP.m2 * parDP.l1 * parDP.a2 * cos(xplus(1)) ^ 2 * cos(xplus(3)) * parDP.m1 * parDP.a1 * u - parDP.m2 * parDP.l1 * parDP.a2 * cos(xplus(1)) * cos(xplus(3)) * parDP.m1 * parDP.a1 * sin(xplus(1)) * xplus(2) * xplus(6) - parDP.m2 * parDP.l1 * parDP.a2 * sin(xplus(1)) ^ 2 * sin(xplus(3)) * parDP.m1 * parDP.g * parDP.a1 - parDP.m2 ^ 2 * parDP.l1 ^ 2 * parDP.a2 * cos(xplus(1)) * cos(xplus(3)) * sin(xplus(1)) * xplus(2) * xplus(6) - parDP.m2 * parDP.l1 * parDP.a2 * cos(xplus(1)) * cos(xplus(3)) * parDP.m1 * parDP.g * parDP.a1 * sin(xplus(1)) - parDP.m2 * parDP.l1 * parDP.a2 * sin(xplus(1)) * sin(xplus(3)) * parDP.m1 * parDP.a1 * cos(xplus(1)) * u - parDP.m2 * parDP.l1 * parDP.a2 * sin(xplus(1)) ^ 2 * sin(xplus(3)) * parDP.m1 * parDP.a1 * xplus(2) * xplus(6) - parDP.m2 * parDP.a2 * sin(xplus(3)) * xplus(4) * parDP.l1 * cos(xplus(1)) * xplus(2) * parDP.J1 - parDP.m2 * parDP.a2 * sin(xplus(3)) * xplus(4) * parDP.l1 * cos(xplus(1)) * xplus(2) * parDP.a1 ^ 2 * parDP.m1 + parDP.m2 * parDP.a2 * cos(xplus(3)) * xplus(4) * parDP.l1 * sin(xplus(1)) * xplus(2) * parDP.J1 + parDP.m2 * parDP.a2 * cos(xplus(3)) * xplus(4) * parDP.l1 * sin(xplus(1)) * xplus(2) * parDP.a1 ^ 2 * parDP.m1) / (parDP.J1 * parDP.m2 * parDP.a2 ^ 2 + parDP.J1 * parDP.J2 + parDP.a1 ^ 2 * parDP.m1 * parDP.m2 * parDP.a2 ^ 2 + parDP.a1 ^ 2 * parDP.m1 * parDP.J2 + parDP.m2 ^ 2 * parDP.l1 ^ 2 * parDP.a2 ^ 2 + parDP.m2 * parDP.l1 ^ 2 * parDP.J2 - parDP.m2 ^ 2 * parDP.l1 ^ 2 * parDP.a2 ^ 2 * cos(xplus(1)) ^ 2 * cos(xplus(3)) ^ 2 - 0.2e1 * parDP.m2 ^ 2 * parDP.l1 ^ 2 * parDP.a2 ^ 2 * cos(xplus(1)) * cos(xplus(3)) * sin(xplus(1)) * sin(xplus(3)) - parDP.m2 ^ 2 * parDP.l1 ^ 2 * parDP.a2 ^ 2 * sin(xplus(1)) ^ 2 * sin(xplus(3)) ^ 2) ^ 2 * (0.2e1 * parDP.m2 ^ 2 * parDP.l1 ^ 2 * parDP.a2 ^ 2 * cos(xplus(1)) * cos(xplus(3)) ^ 2 * sin(xplus(1)) + 0.2e1 * parDP.m2 ^ 2 * parDP.l1 ^ 2 * parDP.a2 ^ 2 * sin(xplus(1)) ^ 2 * cos(xplus(3)) * sin(xplus(3)) - 0.2e1 * parDP.m2 ^ 2 * parDP.l1 ^ 2 * parDP.a2 ^ 2 * cos(xplus(1)) ^ 2 * cos(xplus(3)) * sin(xplus(3)) - 0.2e1 * parDP.m2 ^ 2 * parDP.l1 ^ 2 * parDP.a2 ^ 2 * sin(xplus(1)) * sin(xplus(3)) ^ 2 * cos(xplus(1))) (parDP.d2 * parDP.m2 * parDP.l1 ^ 2 + parDP.d2 * parDP.a1 ^ 2 * parDP.m1 - parDP.m2 ^ 2 * parDP.a2 * sin(xplus(3)) * xplus(4) * parDP.l1 ^ 3 * cos(xplus(1)) + parDP.m2 * parDP.l1 * parDP.a2 * cos(xplus(1)) * cos(xplus(3)) * parDP.d2 + parDP.m2 * parDP.l1 * parDP.a2 * sin(xplus(1)) * sin(xplus(3)) * parDP.d2 + parDP.m2 * parDP.l1 * parDP.a2 * cos(xplus(1)) * cos(xplus(3)) * parDP.d1 + parDP.m2 * parDP.l1 * parDP.a2 * sin(xplus(1)) * sin(xplus(3)) * parDP.d1 + parDP.m2 ^ 2 * parDP.a2 * cos(xplus(3)) * xplus(4) * parDP.l1 ^ 3 * sin(xplus(1)) - parDP.m2 ^ 2 * parDP.l1 ^ 2 * parDP.a2 * sin(xplus(1)) ^ 2 * sin(xplus(3)) * xplus(6) + parDP.d2 * parDP.J1 - parDP.m2 ^ 2 * parDP.l1 ^ 2 * parDP.a2 ^ 2 * cos(xplus(1)) ^ 2 * cos(xplus(3)) * sin(xplus(3)) * xplus(4) - parDP.m2 ^ 2 * parDP.l1 ^ 2 * parDP.a2 ^ 2 * sin(xplus(1)) * sin(xplus(3)) ^ 2 * xplus(4) * cos(xplus(1)) + parDP.m2 ^ 2 * parDP.l1 ^ 2 * parDP.a2 ^ 2 * sin(xplus(1)) ^ 2 * sin(xplus(3)) * cos(xplus(3)) * xplus(4) + parDP.m2 ^ 2 * parDP.l1 ^ 2 * parDP.a2 ^ 2 * cos(xplus(1)) * cos(xplus(3)) ^ 2 * xplus(4) * sin(xplus(1)) - parDP.m2 * parDP.l1 * parDP.a2 * cos(xplus(1)) * cos(xplus(3)) * parDP.m1 * parDP.a1 * sin(xplus(1)) * xplus(6) - parDP.m2 ^ 2 * parDP.l1 ^ 2 * parDP.a2 * cos(xplus(1)) * cos(xplus(3)) * sin(xplus(1)) * xplus(6) - parDP.m2 * parDP.l1 * parDP.a2 * sin(xplus(1)) ^ 2 * sin(xplus(3)) * parDP.m1 * parDP.a1 * xplus(6) - parDP.m2 * parDP.a2 * sin(xplus(3)) * xplus(4) * parDP.l1 * cos(xplus(1)) * parDP.J1 - parDP.m2 * parDP.a2 * sin(xplus(3)) * xplus(4) * parDP.l1 * cos(xplus(1)) * parDP.a1 ^ 2 * parDP.m1 + parDP.m2 * parDP.a2 * cos(xplus(3)) * xplus(4) * parDP.l1 * sin(xplus(1)) * parDP.J1 + parDP.m2 * parDP.a2 * cos(xplus(3)) * xplus(4) * parDP.l1 * sin(xplus(1)) * parDP.a1 ^ 2 * parDP.m1) / (parDP.J1 * parDP.m2 * parDP.a2 ^ 2 + parDP.J1 * parDP.J2 + parDP.a1 ^ 2 * parDP.m1 * parDP.m2 * parDP.a2 ^ 2 + parDP.a1 ^ 2 * parDP.m1 * parDP.J2 + parDP.m2 ^ 2 * parDP.l1 ^ 2 * parDP.a2 ^ 2 + parDP.m2 * parDP.l1 ^ 2 * parDP.J2 - parDP.m2 ^ 2 * parDP.l1 ^ 2 * parDP.a2 ^ 2 * cos(xplus(1)) ^ 2 * cos(xplus(3)) ^ 2 - 0.2e1 * parDP.m2 ^ 2 * parDP.l1 ^ 2 * parDP.a2 ^ 2 * cos(xplus(1)) * cos(xplus(3)) * sin(xplus(1)) * sin(xplus(3)) - parDP.m2 ^ 2 * parDP.l1 ^ 2 * parDP.a2 ^ 2 * sin(xplus(1)) ^ 2 * sin(xplus(3)) ^ 2) (-parDP.m2 * parDP.l1 * parDP.a2 * sin(xplus(1)) * cos(xplus(3)) * parDP.d2 * xplus(4) + parDP.m2 * parDP.l1 * parDP.a2 * sin(xplus(1)) * cos(xplus(3)) * parDP.d2 * xplus(2) + parDP.m2 * parDP.l1 * parDP.a2 * cos(xplus(1)) * sin(xplus(3)) * parDP.d2 * xplus(4) - parDP.m2 * parDP.l1 * parDP.a2 * cos(xplus(1)) * sin(xplus(3)) * parDP.d2 * xplus(2) - parDP.m2 ^ 2 * parDP.l1 ^ 2 * parDP.a2 ^ 2 * sin(xplus(1)) ^ 2 * sin(xplus(3)) ^ 2 * xplus(4) * xplus(2) + parDP.m2 ^ 2 * parDP.l1 ^ 2 * parDP.a2 ^ 2 * sin(xplus(1)) ^ 2 * cos(xplus(3)) ^ 2 * xplus(4) * xplus(2) - 0.4e1 * parDP.m2 ^ 2 * parDP.l1 ^ 2 * parDP.a2 ^ 2 * cos(xplus(1)) * cos(xplus(3)) * sin(xplus(3)) * xplus(4) * xplus(2) * sin(xplus(1)) + parDP.m2 ^ 2 * parDP.l1 ^ 2 * parDP.a2 ^ 2 * cos(xplus(1)) ^ 2 * sin(xplus(3)) ^ 2 * xplus(4) * xplus(2) - parDP.m2 ^ 2 * parDP.l1 ^ 2 * parDP.a2 ^ 2 * cos(xplus(1)) ^ 2 * cos(xplus(3)) ^ 2 * xplus(4) * xplus(2) - parDP.m2 ^ 2 * parDP.a2 * sin(xplus(3)) * u * parDP.l1 ^ 2 - parDP.m2 ^ 2 * parDP.a2 * sin(xplus(3)) * xplus(4) * parDP.l1 ^ 3 * sin(xplus(1)) * xplus(2) + parDP.m2 * parDP.l1 * parDP.a2 * sin(xplus(1)) * cos(xplus(3)) * parDP.d1 * xplus(2) - parDP.m2 * parDP.l1 * parDP.a2 * cos(xplus(1)) * sin(xplus(3)) * parDP.d1 * xplus(2) + parDP.m2 ^ 2 * parDP.l1 ^ 2 * parDP.a2 * cos(xplus(1)) ^ 2 * sin(xplus(3)) * u - parDP.m2 ^ 2 * parDP.a2 * cos(xplus(3)) * xplus(4) * parDP.l1 ^ 3 * cos(xplus(1)) * xplus(2) + parDP.m2 ^ 2 * parDP.l1 ^ 2 * parDP.a2 * sin(xplus(1)) * sin(xplus(3)) * parDP.g * cos(xplus(1)) - parDP.m2 ^ 2 * parDP.l1 ^ 2 * parDP.a2 * cos(xplus(1)) * cos(xplus(3)) * u * sin(xplus(1)) + parDP.m2 ^ 2 * parDP.g * parDP.a2 * cos(xplus(3)) * parDP.l1 ^ 2 + parDP.m2 * parDP.a2 * cos(xplus(3)) * xplus(4) * xplus(6) * parDP.a1 ^ 2 * parDP.m1 - parDP.m2 ^ 2 * parDP.l1 ^ 2 * parDP.a2 * sin(xplus(1)) ^ 2 * cos(xplus(3)) * parDP.g - parDP.m2 * parDP.a2 * sin(xplus(3)) * u * parDP.J1 + parDP.m2 * parDP.g * parDP.a2 * cos(xplus(3)) * parDP.J1 + parDP.m2 ^ 2 * parDP.l1 ^ 2 * parDP.a2 * sin(xplus(1)) * sin(xplus(3)) * xplus(2) * xplus(6) * cos(xplus(1)) + parDP.m2 * parDP.a2 * cos(xplus(3)) * xplus(4) * xplus(6) * parDP.J1 + parDP.m2 ^ 2 * parDP.a2 * cos(xplus(3)) * xplus(4) * xplus(6) * parDP.l1 ^ 2 + parDP.m2 * parDP.g * parDP.a2 * cos(xplus(3)) * parDP.a1 ^ 2 * parDP.m1 - parDP.m2 * parDP.a2 * sin(xplus(3)) * u * parDP.a1 ^ 2 * parDP.m1 - parDP.m2 * parDP.l1 * parDP.a2 * cos(xplus(1)) * cos(xplus(3)) * parDP.m1 * parDP.a1 * u * sin(xplus(1)) - parDP.m2 ^ 2 * parDP.l1 ^ 2 * parDP.a2 * sin(xplus(1)) ^ 2 * cos(xplus(3)) * xplus(2) * xplus(6) - parDP.m2 * parDP.l1 * parDP.a2 * sin(xplus(1)) ^ 2 * cos(xplus(3)) * parDP.m1 * parDP.a1 * xplus(2) * xplus(6) + parDP.m2 * parDP.l1 * parDP.a2 * sin(xplus(1)) * sin(xplus(3)) * parDP.m1 * parDP.g * parDP.a1 * cos(xplus(1)) - parDP.m2 * parDP.l1 * parDP.a2 * sin(xplus(1)) ^ 2 * cos(xplus(3)) * parDP.m1 * parDP.g * parDP.a1 + parDP.m2 * parDP.l1 * parDP.a2 * cos(xplus(1)) ^ 2 * sin(xplus(3)) * parDP.m1 * parDP.a1 * u + parDP.m2 * parDP.l1 * parDP.a2 * sin(xplus(1)) * sin(xplus(3)) * parDP.m1 * parDP.a1 * xplus(2) * xplus(6) * cos(xplus(1)) - parDP.m2 * parDP.a2 * sin(xplus(3)) * xplus(4) * parDP.l1 * sin(xplus(1)) * xplus(2) * parDP.J1 - parDP.m2 * parDP.a2 * sin(xplus(3)) * xplus(4) * parDP.l1 * sin(xplus(1)) * xplus(2) * parDP.a1 ^ 2 * parDP.m1 - parDP.m2 * parDP.a2 * cos(xplus(3)) * xplus(4) * parDP.l1 * cos(xplus(1)) * xplus(2) * parDP.J1 - parDP.m2 * parDP.a2 * cos(xplus(3)) * xplus(4) * parDP.l1 * cos(xplus(1)) * xplus(2) * parDP.a1 ^ 2 * parDP.m1) / (parDP.J1 * parDP.m2 * parDP.a2 ^ 2 + parDP.J1 * parDP.J2 + parDP.a1 ^ 2 * parDP.m1 * parDP.m2 * parDP.a2 ^ 2 + parDP.a1 ^ 2 * parDP.m1 * parDP.J2 + parDP.m2 ^ 2 * parDP.l1 ^ 2 * parDP.a2 ^ 2 + parDP.m2 * parDP.l1 ^ 2 * parDP.J2 - parDP.m2 ^ 2 * parDP.l1 ^ 2 * parDP.a2 ^ 2 * cos(xplus(1)) ^ 2 * cos(xplus(3)) ^ 2 - 0.2e1 * parDP.m2 ^ 2 * parDP.l1 ^ 2 * parDP.a2 ^ 2 * cos(xplus(1)) * cos(xplus(3)) * sin(xplus(1)) * sin(xplus(3)) - parDP.m2 ^ 2 * parDP.l1 ^ 2 * parDP.a2 ^ 2 * sin(xplus(1)) ^ 2 * sin(xplus(3)) ^ 2) - (parDP.d2 * xplus(2) * parDP.m2 * parDP.l1 ^ 2 - parDP.d2 * xplus(4) * parDP.m2 * parDP.l1 ^ 2 - parDP.d2 * xplus(4) * parDP.a1 ^ 2 * parDP.m1 + parDP.d2 * xplus(2) * parDP.a1 ^ 2 * parDP.m1 - parDP.m2 ^ 2 * parDP.a2 * sin(xplus(3)) * xplus(4) * parDP.l1 ^ 3 * cos(xplus(1)) * xplus(2) - parDP.m2 * parDP.l1 * parDP.a2 * cos(xplus(1)) * cos(xplus(3)) * parDP.d2 * xplus(4) + parDP.m2 * parDP.l1 * parDP.a2 * cos(xplus(1)) * cos(xplus(3)) * parDP.d2 * xplus(2) - parDP.m2 * parDP.l1 * parDP.a2 * sin(xplus(1)) * sin(xplus(3)) * parDP.d2 * xplus(4) + parDP.m2 * parDP.l1 * parDP.a2 * sin(xplus(1)) * sin(xplus(3)) * parDP.d2 * xplus(2) + parDP.m2 * parDP.l1 * parDP.a2 * cos(xplus(1)) * cos(xplus(3)) * parDP.d1 * xplus(2) + parDP.m2 * parDP.l1 * parDP.a2 * sin(xplus(1)) * sin(xplus(3)) * parDP.d1 * xplus(2) - parDP.m2 ^ 2 * parDP.l1 ^ 2 * parDP.a2 * cos(xplus(1)) * cos(xplus(3)) * parDP.g * sin(xplus(1)) - parDP.m2 ^ 2 * parDP.l1 ^ 2 * parDP.a2 * sin(xplus(1)) * sin(xplus(3)) * cos(xplus(1)) * u + parDP.m2 ^ 2 * parDP.a2 * cos(xplus(3)) * xplus(4) * parDP.l1 ^ 3 * sin(xplus(1)) * xplus(2) - parDP.m2 ^ 2 * parDP.l1 ^ 2 * parDP.a2 * sin(xplus(1)) ^ 2 * sin(xplus(3)) * xplus(2) * xplus(6) + parDP.m2 * parDP.a2 * sin(xplus(3)) * xplus(4) * xplus(6) * parDP.a1 ^ 2 * parDP.m1 + parDP.m2 ^ 2 * parDP.g * parDP.a2 * sin(xplus(3)) * parDP.l1 ^ 2 + parDP.m2 * parDP.g * parDP.a2 * sin(xplus(3)) * parDP.J1 + parDP.m2 * parDP.a2 * cos(xplus(3)) * u * parDP.J1 + parDP.m2 ^ 2 * parDP.a2 * cos(xplus(3)) * u * parDP.l1 ^ 2 - parDP.m2 ^ 2 * parDP.l1 ^ 2 * parDP.a2 * sin(xplus(1)) ^ 2 * sin(xplus(3)) * parDP.g + parDP.m2 * parDP.a2 * sin(xplus(3)) * xplus(4) * xplus(6) * parDP.J1 + parDP.m2 ^ 2 * parDP.a2 * sin(xplus(3)) * xplus(4) * xplus(6) * parDP.l1 ^ 2 + parDP.m2 * parDP.g * parDP.a2 * sin(xplus(3)) * parDP.a1 ^ 2 * parDP.m1 + parDP.m2 * parDP.a2 * cos(xplus(3)) * u * parDP.a1 ^ 2 * parDP.m1 - parDP.m2 ^ 2 * parDP.l1 ^ 2 * parDP.a2 * cos(xplus(1)) ^ 2 * cos(xplus(3)) * u - parDP.d2 * xplus(4) * parDP.J1 + parDP.d2 * xplus(2) * parDP.J1 - parDP.m2 ^ 2 * parDP.l1 ^ 2 * parDP.a2 ^ 2 * cos(xplus(1)) ^ 2 * cos(xplus(3)) * sin(xplus(3)) * xplus(4) * xplus(2) - parDP.m2 ^ 2 * parDP.l1 ^ 2 * parDP.a2 ^ 2 * sin(xplus(1)) * sin(xplus(3)) ^ 2 * xplus(4) * cos(xplus(1)) * xplus(2) + parDP.m2 ^ 2 * parDP.l1 ^ 2 * parDP.a2 ^ 2 * sin(xplus(1)) ^ 2 * sin(xplus(3)) * cos(xplus(3)) * xplus(4) * xplus(2) + parDP.m2 ^ 2 * parDP.l1 ^ 2 * parDP.a2 ^ 2 * cos(xplus(1)) * cos(xplus(3)) ^ 2 * xplus(4) * sin(xplus(1)) * xplus(2) - parDP.m2 * parDP.l1 * parDP.a2 * cos(xplus(1)) ^ 2 * cos(xplus(3)) * parDP.m1 * parDP.a1 * u - parDP.m2 * parDP.l1 * parDP.a2 * cos(xplus(1)) * cos(xplus(3)) * parDP.m1 * parDP.a1 * sin(xplus(1)) * xplus(2) * xplus(6) - parDP.m2 * parDP.l1 * parDP.a2 * sin(xplus(1)) ^ 2 * sin(xplus(3)) * parDP.m1 * parDP.g * parDP.a1 - parDP.m2 ^ 2 * parDP.l1 ^ 2 * parDP.a2 * cos(xplus(1)) * cos(xplus(3)) * sin(xplus(1)) * xplus(2) * xplus(6) - parDP.m2 * parDP.l1 * parDP.a2 * cos(xplus(1)) * cos(xplus(3)) * parDP.m1 * parDP.g * parDP.a1 * sin(xplus(1)) - parDP.m2 * parDP.l1 * parDP.a2 * sin(xplus(1)) * sin(xplus(3)) * parDP.m1 * parDP.a1 * cos(xplus(1)) * u - parDP.m2 * parDP.l1 * parDP.a2 * sin(xplus(1)) ^ 2 * sin(xplus(3)) * parDP.m1 * parDP.a1 * xplus(2) * xplus(6) - parDP.m2 * parDP.a2 * sin(xplus(3)) * xplus(4) * parDP.l1 * cos(xplus(1)) * xplus(2) * parDP.J1 - parDP.m2 * parDP.a2 * sin(xplus(3)) * xplus(4) * parDP.l1 * cos(xplus(1)) * xplus(2) * parDP.a1 ^ 2 * parDP.m1 + parDP.m2 * parDP.a2 * cos(xplus(3)) * xplus(4) * parDP.l1 * sin(xplus(1)) * xplus(2) * parDP.J1 + parDP.m2 * parDP.a2 * cos(xplus(3)) * xplus(4) * parDP.l1 * sin(xplus(1)) * xplus(2) * parDP.a1 ^ 2 * parDP.m1) / (parDP.J1 * parDP.m2 * parDP.a2 ^ 2 + parDP.J1 * parDP.J2 + parDP.a1 ^ 2 * parDP.m1 * parDP.m2 * parDP.a2 ^ 2 + parDP.a1 ^ 2 * parDP.m1 * parDP.J2 + parDP.m2 ^ 2 * parDP.l1 ^ 2 * parDP.a2 ^ 2 + parDP.m2 * parDP.l1 ^ 2 * parDP.J2 - parDP.m2 ^ 2 * parDP.l1 ^ 2 * parDP.a2 ^ 2 * cos(xplus(1)) ^ 2 * cos(xplus(3)) ^ 2 - 0.2e1 * parDP.m2 ^ 2 * parDP.l1 ^ 2 * parDP.a2 ^ 2 * cos(xplus(1)) * cos(xplus(3)) * sin(xplus(1)) * sin(xplus(3)) - parDP.m2 ^ 2 * parDP.l1 ^ 2 * parDP.a2 ^ 2 * sin(xplus(1)) ^ 2 * sin(xplus(3)) ^ 2) ^ 2 * (0.2e1 * parDP.m2 ^ 2 * parDP.l1 ^ 2 * parDP.a2 ^ 2 * cos(xplus(1)) ^ 2 * cos(xplus(3)) * sin(xplus(3)) + 0.2e1 * parDP.m2 ^ 2 * parDP.l1 ^ 2 * parDP.a2 ^ 2 * sin(xplus(1)) * sin(xplus(3)) ^ 2 * cos(xplus(1)) - 0.2e1 * parDP.m2 ^ 2 * parDP.l1 ^ 2 * parDP.a2 ^ 2 * cos(xplus(1)) * cos(xplus(3)) ^ 2 * sin(xplus(1)) - 0.2e1 * parDP.m2 ^ 2 * parDP.l1 ^ 2 * parDP.a2 ^ 2 * sin(xplus(1)) ^ 2 * cos(xplus(3)) * sin(xplus(3))) (-parDP.d2 * parDP.m2 * parDP.l1 ^ 2 - parDP.d2 * parDP.a1 ^ 2 * parDP.m1 - parDP.m2 ^ 2 * parDP.a2 * sin(xplus(3)) * parDP.l1 ^ 3 * cos(xplus(1)) * xplus(2) - parDP.m2 * parDP.l1 * parDP.a2 * cos(xplus(1)) * cos(xplus(3)) * parDP.d2 - parDP.m2 * parDP.l1 * parDP.a2 * sin(xplus(1)) * sin(xplus(3)) * parDP.d2 + parDP.m2 ^ 2 * parDP.a2 * cos(xplus(3)) * parDP.l1 ^ 3 * sin(xplus(1)) * xplus(2) + parDP.m2 * parDP.a2 * sin(xplus(3)) * xplus(6) * parDP.a1 ^ 2 * parDP.m1 + parDP.m2 * parDP.a2 * sin(xplus(3)) * xplus(6) * parDP.J1 + parDP.m2 ^ 2 * parDP.a2 * sin(xplus(3)) * xplus(6) * parDP.l1 ^ 2 - parDP.d2 * parDP.J1 - parDP.m2 ^ 2 * parDP.l1 ^ 2 * parDP.a2 ^ 2 * cos(xplus(1)) ^ 2 * cos(xplus(3)) * sin(xplus(3)) * xplus(2) - parDP.m2 ^ 2 * parDP.l1 ^ 2 * parDP.a2 ^ 2 * sin(xplus(1)) * sin(xplus(3)) ^ 2 * cos(xplus(1)) * xplus(2) + parDP.m2 ^ 2 * parDP.l1 ^ 2 * parDP.a2 ^ 2 * sin(xplus(1)) ^ 2 * sin(xplus(3)) * cos(xplus(3)) * xplus(2) + parDP.m2 ^ 2 * parDP.l1 ^ 2 * parDP.a2 ^ 2 * cos(xplus(1)) * cos(xplus(3)) ^ 2 * sin(xplus(1)) * xplus(2) - parDP.m2 * parDP.a2 * sin(xplus(3)) * parDP.l1 * cos(xplus(1)) * xplus(2) * parDP.J1 - parDP.m2 * parDP.a2 * sin(xplus(3)) * parDP.l1 * cos(xplus(1)) * xplus(2) * parDP.a1 ^ 2 * parDP.m1 + parDP.m2 * parDP.a2 * cos(xplus(3)) * parDP.l1 * sin(xplus(1)) * xplus(2) * parDP.J1 + parDP.m2 * parDP.a2 * cos(xplus(3)) * parDP.l1 * sin(xplus(1)) * xplus(2) * parDP.a1 ^ 2 * parDP.m1) / (parDP.J1 * parDP.m2 * parDP.a2 ^ 2 + parDP.J1 * parDP.J2 + parDP.a1 ^ 2 * parDP.m1 * parDP.m2 * parDP.a2 ^ 2 + parDP.a1 ^ 2 * parDP.m1 * parDP.J2 + parDP.m2 ^ 2 * parDP.l1 ^ 2 * parDP.a2 ^ 2 + parDP.m2 * parDP.l1 ^ 2 * parDP.J2 - parDP.m2 ^ 2 * parDP.l1 ^ 2 * parDP.a2 ^ 2 * cos(xplus(1)) ^ 2 * cos(xplus(3)) ^ 2 - 0.2e1 * parDP.m2 ^ 2 * parDP.l1 ^ 2 * parDP.a2 ^ 2 * cos(xplus(1)) * cos(xplus(3)) * sin(xplus(1)) * sin(xplus(3)) - parDP.m2 ^ 2 * parDP.l1 ^ 2 * parDP.a2 ^ 2 * sin(xplus(1)) ^ 2 * sin(xplus(3)) ^ 2) 0 (-parDP.m2 ^ 2 * parDP.l1 ^ 2 * parDP.a2 * sin(xplus(1)) ^ 2 * sin(xplus(3)) * xplus(2) + parDP.m2 * parDP.a2 * sin(xplus(3)) * xplus(4) * parDP.a1 ^ 2 * parDP.m1 + parDP.m2 * parDP.a2 * sin(xplus(3)) * xplus(4) * parDP.J1 + parDP.m2 ^ 2 * parDP.a2 * sin(xplus(3)) * xplus(4) * parDP.l1 ^ 2 - parDP.m2 * parDP.l1 * parDP.a2 * cos(xplus(1)) * cos(xplus(3)) * parDP.m1 * parDP.a1 * sin(xplus(1)) * xplus(2) - parDP.m2 ^ 2 * parDP.l1 ^ 2 * parDP.a2 * cos(xplus(1)) * cos(xplus(3)) * sin(xplus(1)) * xplus(2) - parDP.m2 * parDP.l1 * parDP.a2 * sin(xplus(1)) ^ 2 * sin(xplus(3)) * parDP.m1 * parDP.a1 * xplus(2)) / (parDP.J1 * parDP.m2 * parDP.a2 ^ 2 + parDP.J1 * parDP.J2 + parDP.a1 ^ 2 * parDP.m1 * parDP.m2 * parDP.a2 ^ 2 + parDP.a1 ^ 2 * parDP.m1 * parDP.J2 + parDP.m2 ^ 2 * parDP.l1 ^ 2 * parDP.a2 ^ 2 + parDP.m2 * parDP.l1 ^ 2 * parDP.J2 - parDP.m2 ^ 2 * parDP.l1 ^ 2 * parDP.a2 ^ 2 * cos(xplus(1)) ^ 2 * cos(xplus(3)) ^ 2 - 0.2e1 * parDP.m2 ^ 2 * parDP.l1 ^ 2 * parDP.a2 ^ 2 * cos(xplus(1)) * cos(xplus(3)) * sin(xplus(1)) * sin(xplus(3)) - parDP.m2 ^ 2 * parDP.l1 ^ 2 * parDP.a2 ^ 2 * sin(xplus(1)) ^ 2 * sin(xplus(3)) ^ 2)  ;
    0 0 0 0 0 1 ;
    0 0 0 0 0 0;];
end

== matlab function Doppelpendel_EKF_2015a/Vorsteuerung/Trajektorienplanung ==
  settings: updateMethod=DISCRETE  sampleTime=parLQR.Ta
  data: time input; deltax input; Te input; zz output; parFF parameter; uFF output; statesd output; start1 input; reset1 input; start2 input; start output; reset2 input; t output; start3 input; reset3 input
%%%%%%%%%%%%%%%%%%%%%%%%%%%%%%%%%%%%%%%%%%%%%%%%%%%%%%%%%%%%%%%%%%%%%%%%%%%
%
% Trajektorienplanung zum Versetzten des Doppelpendels
%
%%%%%%%%%%%%%%%%%%%%%%%%%%%%%%%%%%%%%%%%%%%%%%%%%%%%%%%%%%%%%%%%%%%%%%%%%%%

function [zz,uFF,statesd,start,t] = Trajektorienplanung(time,deltax,Te,parFF,start1,reset1,start2,reset2,start3,reset3)

persistent tstart
if isempty(tstart) tstart = double(0); end
persistent x0
if isempty(x0) x0 = double(0); end
persistent xT
if isempty(xT) xT = double(deltax); end


if reset1>0.5 || reset2>0.5 || reset3>0.5
    
    tstart = time;

end
%Zeit ab tstart
t = time - tstart;


if  start1>0.5 
    
    start = 1;
    
    if start2<0.5
        
        x0=0;
        xT=deltax; 
        
    else
        
        if start3<0.5
        
            x0=deltax;
            xT=-deltax; 
        
        else
    
            %Anfangs- und Endwert
            x0=-deltax;
            xT=deltax;
            
        end

    end
    
else
    
    start = 0;
    
end

% Folgendes hier bitte ausführen:
% 1.) Umrechnung auf Anfangs- und Endwert des Flachen Ausgangs
% 2.) Funktion Trajektorie() ergänzen
% 3.) Vorsteuerungsberechnung uFF ergänzen
% 4.) Sollzustandsverlauf statesd ergänzen

%p Umrechnung auf Anfangs- und Endwert des Flachen Ausgangs
% parFF.VV = inv(parFF.VVinv);

z0 = parFF.VV(1,5) * x0;
zT = parFF.VV(1,5) * xT;

zz = Trajektorie(start,t,Te,z0,zT,parFF);
%zz=[z,zdot,z2dot,z3dot,z4dot,z5dot,z6dot];

%p Vorsteuerung laut S.27/(2.22)
%p zz (Delta_z) muss zu einem Spaltenvektor gemacht werden
uFF = parFF.aa'*zz';
%p Sollzustandsverlauf
statesd = parFF.VVinv*zz(1:6)';

end

%%%%%%%%%%%%%%%%%%%%%%%%%%%%%%%%%%%%%%%%%%%%%%%%%%%%%%%%%%%%%%%%%%%%%%%%%%    
function [zz] = Trajektorie(start,t,Te,z0,zT,parFF)
    
    if start<0.5

        z     = z0; 
        zdot  = 0; 
        z2dot = 0; 
        z3dot = 0; 
        z4dot = 0; 
        z5dot = 0; 
        z6dot = 0; 

    elseif start>0.5 && t<Te

        % Folgendes hier bitte ausführen:
        % 1.) Berechnung der Solltrajektorie
        beta7 = parFF.beta7/Te^7;
        beta8 = parFF.beta8/Te^8;
        beta9 = parFF.beta9/Te^9;
        beta10 = parFF.beta10/Te^10;
        beta11 = parFF.beta11/Te^11;
        beta12 = parFF.beta12/Te^12;
        beta13 = parFF.beta13/Te^13;
        
        zT_z0 = zT - z0;      
                
        z = z0 + zT_z0 * (beta7 * t.^ 7 + beta8 * t.^ 8 + beta9 * t.^ 9 + beta10 * t.^ 10 + beta11 * t.^ 11 + beta12 * t.^ 12 + beta13 * t.^ 13);
        zdot =  zT_z0 * (7 * beta7 * t.^ 6 + 8 * beta8 * t.^ 7 + 9 * beta9 * t.^ 8 + 10 * beta10 * t.^ 9 + 11 * beta11 * t.^ 10 + 12 * beta12 * t.^ 11 + 13 * beta13 * t.^ 12);
        z2dot = zT_z0 * (42 * beta7 * t.^ 5 + 56 * beta8 * t.^ 6 + 72 * beta9 * t.^ 7 + 90 * beta10 * t.^ 8 + 110 * beta11 * t.^ 9 + 132 * beta12 * t.^ 10 + 156 * beta13 * t.^ 11);
        z3dot = zT_z0 * (210 * beta7 * t.^ 4 + 336 * beta8 * t.^ 5 + 504 * beta9 * t.^ 6 + 720 * beta10 * t.^ 7 + 990 * beta11 * t.^ 8 + 1320 * beta12 * t.^ 9 + 1716 * beta13 * t.^ 10);
        z4dot = zT_z0 * (840 * beta7 * t.^ 3 + 1680 * beta8 * t.^ 4 + 3024 * beta9 * t.^ 5 + 5040 * beta10 * t.^ 6 + 7920 * beta11 * t.^ 7 + 11880 * beta12 * t.^ 8 + 17160 * beta13 * t.^ 9);
        z5dot = zT_z0 * (2520 * beta7 * t.^ 2 + 6720 * beta8 * t.^ 3 + 15120 * beta9 * t.^ 4 + 30240 * beta10 * t.^ 5 + 55440 * beta11 * t.^ 6 + 95040 * beta12 * t.^ 7 + 154440 * beta13 * t.^ 8);
        z6dot = zT_z0 * (5040 * beta7 * t + 20160 * beta8 * t.^ 2 + 60480 * beta9 * t.^ 3 + 151200 * beta10 * t.^ 4 + 332640 * beta11 * t.^ 5 + 665280 * beta12 * t.^ 6 + 1235520 * beta13 * t.^ 7);


    else

        z     = zT; 
        zdot  = 0; 
        z2dot = 0; 
        z3dot = 0; 
        z4dot = 0; 
        z5dot = 0; 
        z6dot = 0; 

    end

    zz=[z,zdot,z2dot,z3dot,z4dot,z5dot,z6dot];

end
